simulink model "controller_AWBT"  (R2015a)
settings: Solver=ode5  StartTime=0.0  StopTime=9  FixedStep=1e-4  RelTol=1e-3
values from neighbouring files (symbols this model uses):
  Ap = A    [main_matlab_version_4.m]    (also in plant.mat = [-0.773996386153 -96.4009703983 0 0 96.979553948 -1.63547954)
  Bp = B    [main_matlab_version_4.m]    (also in plant.mat = [-0.230745598618  -0.153904745996; 0.0612777559553  0.060617)
  Cp = C    [main_matlab_version_4.m]    (also in plant.mat = [-23.1554338545 9.56281796835 0.435674513054 -0.46619419818])
  Hp = E    [main_matlab_version_4.m]    (also in plant.mat = [0.258916103899 0.10195659276 -1.80129126805 -4.56185147008])
  Lambda = [5.58858586263e-05  0.000107348957209; 5.1607851515e-05  9.34227642014e-05; -0.000303330434435  -0.000279469710906; -0.00200633369332  -0.00367108921652; -0.999913291495  0.000114263611536; 0.000204848209343  -0.999721959339]    [controller_khat.mat]
libraries: cstblocks x2, simulink x1
settings Model: Creator=p4wp4w  LastModifiedBy=p4wp4w
settings SolverCC: AlgebraicLoopSolver=LineSearch

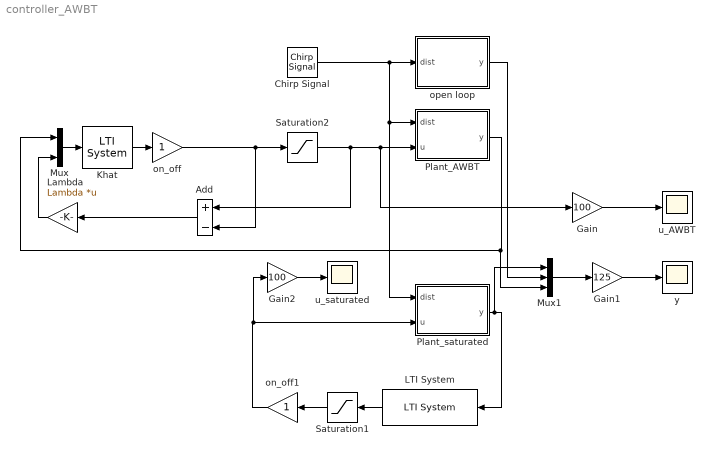
== system controller_AWBT ==
  Add : Sum  Inputs=+-
  Chirp Signal : simulink/Sources/Chirp Signal  f1=0.1  T=9  f2=90
  Gain : Gain  Gain=100
  Gain1 : Gain  Gain=125
  Gain2 : Gain  Gain=100
  Khat : cstblocks/LTI System  sys=Khat  IC=[]
  LTI System : cstblocks/LTI System  sys=controller_implemented  IC=[]
  Lambda : Gain  Gain=Lambda  Multiplication=Matrix(K*u)
  Mux : Mux  Inputs=2
  Mux1 : Mux  Inputs=3
  Plant_AWBT : Subsystem
  Plant_saturated : Subsystem
  Saturation1 : Saturate  UpperLimit=2  LowerLimit=-2
  Saturation2 : Saturate  UpperLimit=2  LowerLimit=-2
  on_off : Gain
  on_off1 : Gain
  open loop : Subsystem
  u_AWBT : Scope
      settings: YMin=-0.75  YMax=0.75
  u_saturated : Scope
      settings: SaveName=ScopeData2
  y : Scope
      settings: ShowLegends=on  YMin=-4  YMax=4
  wires:
  Mux/1 -> Khat/1
  Plant_AWBT/1(y) -> Mux1/3, Mux/1
  Khat/1 -> on_off/1
  Chirp Signal/1 -> open loop/1(dist), Plant_saturated/1(dist), Plant_AWBT/1(dist)
  LTI System/1 -> Saturation1/1
  Plant_saturated/1(y) -> LTI System/1, Mux1/1
  Saturation1/1 -> on_off1/1
  Mux1/1 -> Gain1/1
  open loop/1(y) -> Mux1/2
  on_off1/1 -> Gain2/1, Plant_saturated/2(u)
  Lambda/1 -> Mux/2
  on_off/1 -> Add/2, Saturation2/1
  Saturation2/1 -> Add/1, Gain/1, Plant_AWBT/2(u)
  Add/1 -> Lambda/1
  Gain/1 -> u_AWBT/1
  Gain1/1 -> y/1
  Gain2/1 -> u_saturated/1

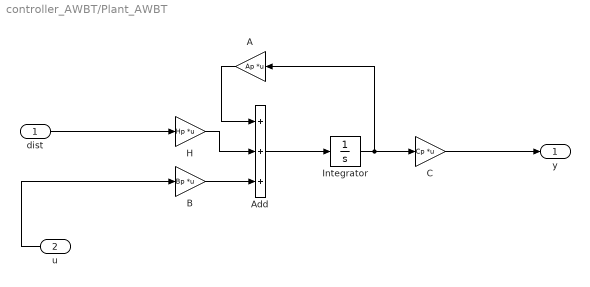
== system controller_AWBT/Plant_AWBT ==
  dist : Inport
  u : Inport  Port=2
  A : Gain  Gain=Ap  Multiplication=Matrix(K*u)
  Add : Sum  Inputs=+++
  B : Gain  Gain=Bp  Multiplication=Matrix(K*u)
  C : Gain  Gain=Cp  Multiplication=Matrix(K*u)
  H : Gain  Gain=Hp  Multiplication=Matrix(K*u)
  Integrator : Integrator
  y : Outport
  wires:
  Add/1 -> Integrator/1
  H/1 -> Add/2
  A/1 -> Add/1
  dist/1 -> H/1
  B/1 -> Add/3
  Integrator/1 -> C/1, A/1
  u/1 -> B/1
  C/1 -> y/1

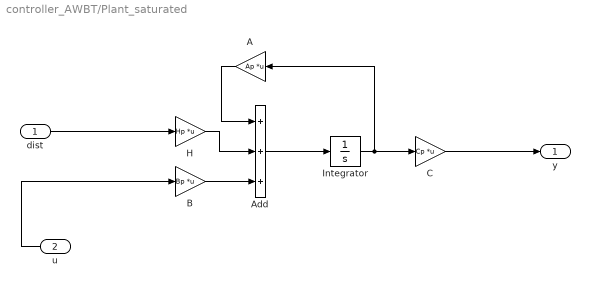
== system controller_AWBT/Plant_saturated ==
  dist : Inport
  u : Inport  Port=2
  A : Gain  Gain=Ap  Multiplication=Matrix(K*u)
  Add : Sum  Inputs=+++
  B : Gain  Gain=Bp  Multiplication=Matrix(K*u)
  C : Gain  Gain=Cp  Multiplication=Matrix(K*u)
  H : Gain  Gain=Hp  Multiplication=Matrix(K*u)
  Integrator : Integrator
  y : Outport
  wires:
  u/1 -> B/1
  Integrator/1 -> A/1, C/1
  B/1 -> Add/3
  dist/1 -> H/1
  A/1 -> Add/1
  H/1 -> Add/2
  Add/1 -> Integrator/1
  C/1 -> y/1

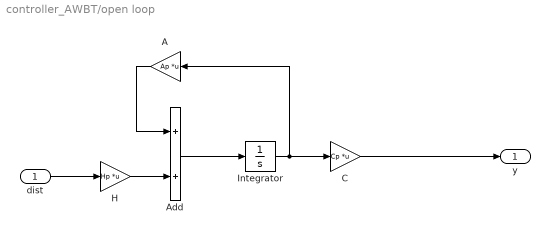
== system controller_AWBT/open loop ==
  dist : Inport
  A : Gain  Gain=Ap  Multiplication=Matrix(K*u)
  Add : Sum
  C : Gain  Gain=Cp  Multiplication=Matrix(K*u)
  H : Gain  Gain=Hp  Multiplication=Matrix(K*u)
  Integrator : Integrator
  y : Outport
  wires:
  Integrator/1 -> A/1, C/1
  dist/1 -> H/1
  A/1 -> Add/1
  H/1 -> Add/2
  Add/1 -> Integrator/1
  C/1 -> y/1
